simulink model "ckl_08022311_7_24"  (R2022b)
settings: Solver=VariableStepAuto  StartTime=0.0  StopTime=10.0  RelTol=1e-3
settings Model: Creator=ASUS  LastModifiedBy=ASUS

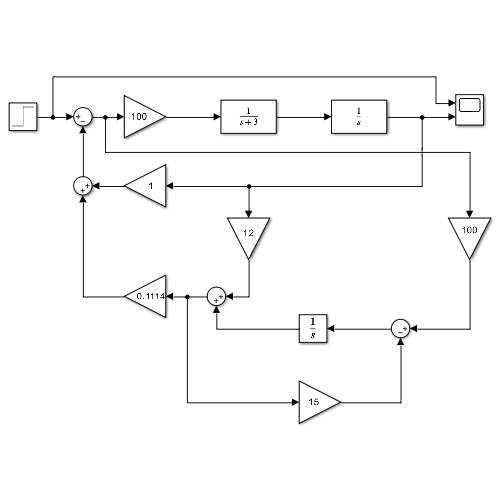
[thumbnail: Simulink's stored preview of the top-level diagram]
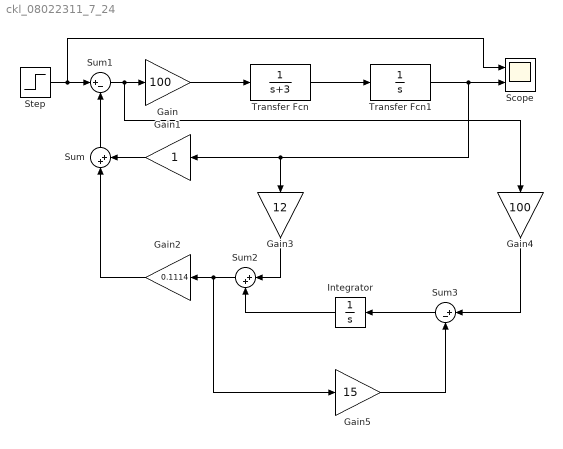
== system ckl_08022311_7_24 ==
  Gain : Gain  Gain=100
  Gain1 : Gain
  Gain2 : Gain  Gain=0.1114
  Gain3 : Gain  Gain=12
  Gain4 : Gain  Gain=100
  Gain5 : Gain  Gain=15
  Integrator : Integrator
  Scope : Scope  NumInputPorts=2
  Step : Step  SampleTime=0
  Sum : Sum  Inputs=|++
  Sum1 : Sum  Inputs=|+-
  Sum2 : Sum  Inputs=|++
  Sum3 : Sum  Inputs=|+-
  Transfer Fcn : TransferFcn  Denominator=[1 3]
  Transfer Fcn1 : TransferFcn  Denominator=[1 0]
  wires:
  Gain/1 -> Transfer Fcn/1
  Transfer Fcn/1 -> Transfer Fcn1/1
  Transfer Fcn1/1 -> Scope/2, Gain3/1, Gain1/1
  Sum1/1 -> Gain4/1, Gain/1
  Step/1 -> Scope/1, Sum1/1
  Sum/1 -> Sum1/2
  Gain1/1 -> Sum/2
  Gain2/1 -> Sum/1
  Sum2/1 -> Gain5/1, Gain2/1
  Gain3/1 -> Sum2/1
  Gain4/1 -> Sum3/1
  Sum3/1 -> Integrator/1
  Gain5/1 -> Sum3/2
  Integrator/1 -> Sum2/2
